simulink model "model_bf_po"  (Simulink 7.0)
settings: Solver=ode45  StartTime=0.0  StopTime=10.0  RelTol=1e-3
libraries: cstblocks x10
settings Model: Creator=fromion  LastModifiedBy=vfromion  ExtModeTrigMode=oneshot  ExtModeArmWhenConnect=off  ExtModeAutoUpdateStatusClock=off
settings DataIOCC: LimitDataPoints=off
settings OptimizationCC: BlockReduction=off  BooleanDataType=off
settings DebuggingCC: SaveWithParameterizedLinksMsg=none  SignalResolutionControl=TryResolveAllWithWarning  SolverPrmCheckMsg=none  MultiTaskDSMMsg=warning  MultiTaskCondExecSysMsg=none  StrictBusMsg=None
settings HardwareCC: TargetUnknown=on
settings RTWCC: IncludeERTFirstTime=on
settings GRTTargetCC: ModelReferenceCompliant=off  CompOptLevelCompliant=off  MatFileLogging=off

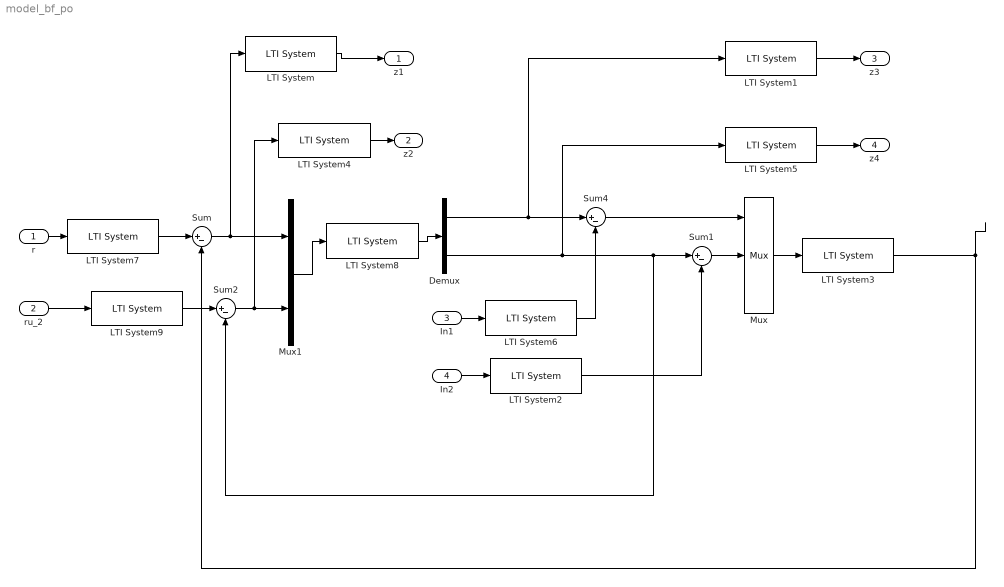
== system model_bf_po ==
  r : Inport
  ru_2 : Inport  Port=2
  In1 : Inport  Port=3
  In2 : Inport  Port=4
  Demux : Demux  Outputs=2
  LTI System : cstblocks/LTI System  SystemSampleTime=-1  sys=W11  IC=0
  LTI System1 : cstblocks/LTI System  SystemSampleTime=-1  sys=W21  IC=0
  LTI System2 : cstblocks/LTI System  SystemSampleTime=-1  sys=Wp2  IC=0
  LTI System3 : cstblocks/LTI System  SystemSampleTime=-1  sys=sys_synt_ss  IC=0
  LTI System4 : cstblocks/LTI System  SystemSampleTime=-1  sys=W12  IC=0
  LTI System5 : cstblocks/LTI System  SystemSampleTime=-1  sys=W22  IC=0
  LTI System6 : cstblocks/LTI System  SystemSampleTime=-1  sys=Wp1  IC=0
  LTI System7 : cstblocks/LTI System  SystemSampleTime=-1  sys=Wpe1  IC=0
  LTI System8 : cstblocks/LTI System  SystemSampleTime=-1  sys=K_hinf_ss  IC=0
  LTI System9 : cstblocks/LTI System  SystemSampleTime=-1  sys=Wpe2  IC=0
  Mux : Mux  Inputs=3
  Mux1 : Mux  Inputs=2
  Sum{,1..2,4} (4 alike) : Sum  Inputs=|+-  SaturateOnIntegerOverflow=on  InputSameDT=on
  z1 : Outport
  z2 : Outport  Port=2
  z3 : Outport  Port=3
  z4 : Outport  Port=4
  wires:
  Sum/1 -> LTI System/1, Mux1/1
  LTI System1/1 -> z3/1
  In1/1 -> LTI System6/1
  r/1 -> LTI System7/1
  LTI System/1 -> z1/1
  LTI System3/1 -> Sum/2
  Sum4/1 -> Mux/1
  Demux/2 -> LTI System5/1, Sum1/1, Sum2/2
  Sum1/1 -> Mux/2
  LTI System5/1 -> z4/1
  LTI System6/1 -> Sum4/2
  In2/1 -> LTI System2/1
  LTI System2/1 -> Sum1/2
  ru_2/1 -> LTI System9/1
  Sum2/1 -> LTI System4/1, Mux1/2
  LTI System4/1 -> z2/1
  Mux/1 -> LTI System3/1
  Demux/1 -> Sum4/1, LTI System1/1
  Mux1/1 -> LTI System8/1
  LTI System8/1 -> Demux/1
  LTI System7/1 -> Sum/1
  LTI System9/1 -> Sum2/1
